simulink model "Quad_Tilt_Rotor_IdealModel"  (R2021b)
settings: Solver=FixedStepAuto  StartTime=0.0  StopTime=6  FixedStep=0.0001  RelTol=1e-3
values from neighbouring files (symbols this model uses):
  desired_initial_orientation = initial_orientation    [parameters_setting_Ideal.m]
  g = 9.8    [parameters_setting_Ideal.m]
  IB = [ 2.237568e-3  0               0 ... (first row only)    [parameters_setting_Ideal.m]
  initial_omega1 = initial_angular_vel1 * abs(initial_angular_vel1)    [parameters_setting_Ideal.m]
  initial_omega2 = initial_angular_vel2 * abs(initial_angular_vel2)    [parameters_setting_Ideal.m]
  initial_omega3 = initial_angular_vel3 * abs(initial_angular_vel3)    [parameters_setting_Ideal.m]
  initial_omega4 = initial_angular_vel4 * abs(initial_angular_vel4)    [parameters_setting_Ideal.m]
  initial_orientation = [ 1 0 0; 0 1 0; 0 0 1 ]    [parameters_setting_Ideal.m]
  Kf = 8.048e-6    (= 8.048e-06)    [parameters_setting_Ideal.m]
  Km = 2.423e-7    (= 2.423e-07)    [parameters_setting_Ideal.m]
  L = 0.1785    [parameters_setting_Ideal.m]
  lower_dalpha = -inf    [parameters_setting_Ideal.m]
  m = 0.429    [parameters_setting_Ideal.m]
  upper_dalpha = inf    [parameters_setting_Ideal.m]
libraries: vrlib x4, sharedutil x1, aerolibutil x1
settings Model: Creator=lucid  LastModifiedBy=lucid

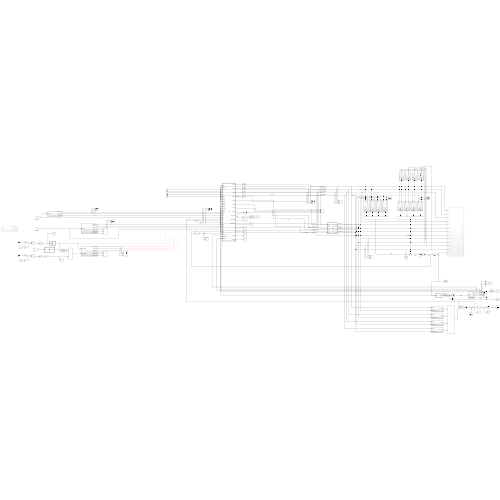
[thumbnail: Simulink's stored preview of the top-level diagram]
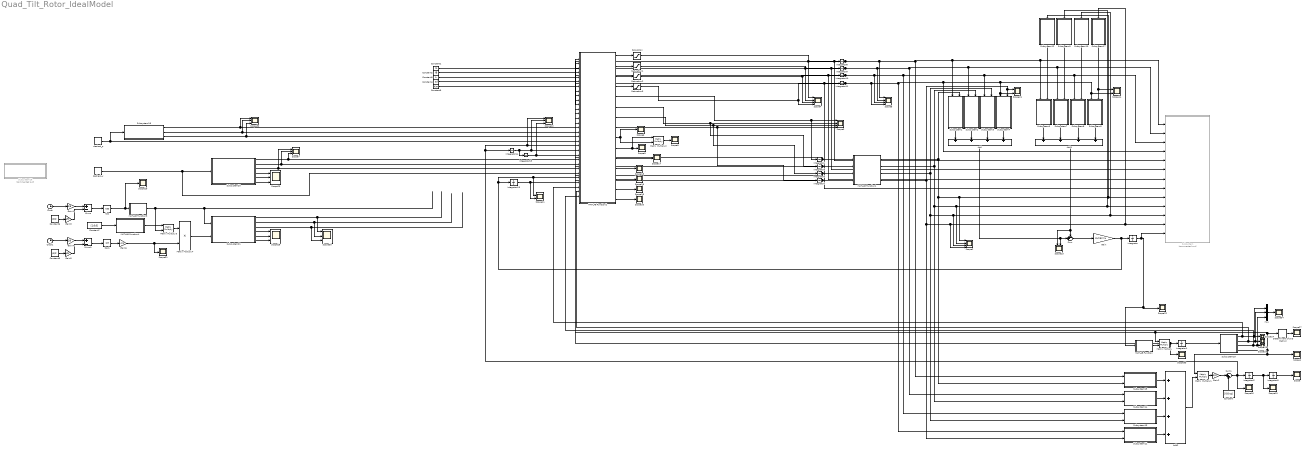
== system Quad_Tilt_Rotor_IdealModel ==
  Add : Sum  Inputs=++++
  Add1 : Sum  Inputs=++++
  Add2 : Sum  Inputs=++++
  Clock : Clock
  Clock1 : Clock
  Constant : Constant  Value=[0;0;-g]
  Constant1 : Constant  Value=m
  Constant2 : Constant  Value=IB
  Constant3 : Constant  Value=L
  Constant4 : Constant  Value=Kf
  Constant5 : Constant  Value=Km
  Constant6 : Constant  Value=pi/2
  Constant7 : Constant  Value=[1;0;0]
  Constant8 : Constant  Value=pi/2
  Cos : Trigonometry  Operator=cos
  Cos1 : Trigonometry
  Determinant of 3x3 Matrix2 : sharedutil/Determinant of 3x3 Matrix  aMode=aMode
      settings: SourceProductBaseCode=AE,PW,DR,MT,UV,VE
  Gain : Gain  Gain=inv(IB)  Multiplication=Matrix(K*u) (u vector)
  Gain{1,3..5} (4 alike) : Gain  Gain=1/6
  Gain2 : Gain  Gain=1/m
  Gain6 : Gain  Gain=-1/6
  Integrator{,2..3,8..11,13..15} (10 alike) : Integrator
  Integrator1 : Integrator  InitialCondition=initial_orientation
  Integrator4 : Integrator  InitialCondition=initial_omega1
  Integrator5 : Integrator  InitialCondition=initial_omega2
  Integrator6 : Integrator  InitialCondition=initial_omega3
  Integrator7 : Integrator  InitialCondition=initial_omega4
  MATLAB Function : MATLAB Function  TreatAsAtomicUnit=on
  MATLAB Function1 : MATLAB Function  TreatAsAtomicUnit=on
  MATLAB Function2 : MATLAB Function  TreatAsAtomicUnit=on
  MATLAB Function3 : MATLAB Function  TreatAsAtomicUnit=on
  MATLAB Function4 : MATLAB Function  TreatAsAtomicUnit=on
  Matrix Multiply{,1..3} (4 alike) : Product  Multiplication=Matrix(*)
  Matrix Multiply4 : Product
  Minus : Sum  Inputs=+-
  Minus1 : Sum  Inputs=+-
  Mux : Mux  Inputs=3
  Saturation{,1..3} (4 alike) : Saturate  UpperLimit=upper_dalpha  LowerLimit=lower_dalpha
  Scope{,1,6,8..10,15..20,22,24..27,29,31,33..34} (21 alike) : Scope
  Scope{11,13..14,21} (4 alike) : Scope  NumInputPorts=2
  Scope{7,12,23,28,30,32} (6 alike) : Scope  NumInputPorts=3
  Scope{2..5} (4 alike) : Scope  NumInputPorts=4
  Subsystem : Subsystem  Commented=on
  Subsystem1 : Subsystem
  Subsystem10 : Subsystem
  Subsystem11 : Subsystem
  Subsystem12 : Subsystem
  Subsystem13 : Subsystem
  Subsystem14 : Subsystem
  Subsystem15 : Subsystem
  Subsystem16 : Subsystem  Commented=on
  Subsystem17 : Subsystem
  Subsystem18 : Subsystem
  Subsystem19 : Subsystem
  Subsystem2 : Subsystem
  Subsystem20 : Subsystem
  Subsystem21 : Subsystem
  Subsystem3 : Subsystem
  Subsystem4 : Subsystem
  Subsystem5 : Subsystem
  Subsystem6 : Subsystem
  Subsystem7 : Subsystem
  Subsystem8 : Subsystem
  Subsystem9 : Subsystem
  Sum : Sum  Inputs=-+|
  Sum1 : Sum  Inputs=|++
  desired_p : Constant  Value=[0;0;0]
  desired_w : Constant  Value=[0;0;0]
  wires:
  Gain/1 -> Integrator13/1, Scope11/1, MATLAB Function2/27(dwB), Integrator/1  "dwB"
  Sum/1 -> Gain/1  "IB*dwB"
  Add/1 -> Scope13/2, Sum/2  "tauB"
  Add1/1 -> Sum/1, Scope13/1  "sumBtauP"
  Integrator/1 -> Subsystem/13(wB), MATLAB Function/1(w), Scope22/1  "wB"
  Subsystem1/1(tauB1) -> Add/1
  Subsystem2/1(tauB2) -> Add/2
  Subsystem3/1(tauB3) -> Add/3
  Subsystem4/1(tauB4) -> Add/4
  Subsystem5/1(BtauP4) -> Add1/4
  Subsystem6/1(BtauP1) -> Add1/1
  Subsystem7/1(BtauP2) -> Add1/2
  Subsystem8/1(BtauP3) -> Add1/3
  Subsystem17/1(tauP4) -> Subsystem5/2(tauP4), Scope14/1
  Subsystem12/1(tauP1) -> Subsystem6/2(tauP1)
  Subsystem9/1(tauP2) -> Subsystem7/2(tauP2)
  Subsystem10/1(tauP3) -> Subsystem8/2(tauP3)
  Integrator8/1 -> Scope5/1, Subsystem6/1(alpha1), Subsystem/1(alpha1), Subsystem1/1(alpha1), Subsystem15/1(alpha1), MATLAB Function2/8(alpha1)  "alpha1"
  Integrator9/1 -> Scope5/2, Subsystem7/1(alpha2), Subsystem/2(alpha2), Subsystem2/1(alpha2), Subsystem14/1(alpha2), MATLAB Function2/9(alpha2)  "alpha2"
  Integrator10/1 -> Scope5/3, Subsystem13/1(alpha3), Subsystem8/1(alpha3), Subsystem/3(alpha3), Subsystem3/1(alpha3), MATLAB Function2/10(alpha3)  "alpha3"
  Integrator11/1 -> Scope5/4, Scope14/2, Subsystem5/1(alpha4), Scope21/2, Subsystem4/1(alpha4), Subsystem/4(alpha4), Subsystem11/1(alpha4), MATLAB Function2/11(alpha4)  "alpha4"
  MATLAB Function1/1(angular_vel1) -> Subsystem15/2(angular_vel1), Scope2/1, Subsystem/9(angular_vel1), Subsystem12/1(Angular_vel1), Subsystem1/2(angular_vel1)  "angular_vel1"
  MATLAB Function1/2(angular_vel2) -> Subsystem14/2(angular_vel2), Scope2/2, Subsystem/10(angular_vel2), Subsystem9/1(Angular_vel2), Subsystem2/2(angular_vel2)  "angular_vel2"
  MATLAB Function1/3(angular_vel3) -> Subsystem13/2(angular_vel3), Scope2/3, Subsystem10/1(Angular_vel3), Subsystem/11(angular_vel3), Subsystem3/2(angular_vel3)  "angular_vel3"
  MATLAB Function1/4(angular_vel4) -> Subsystem11/2(angular_vel4), Scope2/4, Subsystem17/1(Angular_vel4), Subsystem/12(angular_vel4), Scope21/1, Subsystem4/2(angular_vel4)  "angular_vel4"
  Constant/1 -> Sum1/2
  Gain2/1 -> Sum1/1
  Integrator1/1 -> Subsystem19/1(WRB)  "WRB"
  Matrix Multiply/1 -> Scope33/1, Integrator1/1, MATLAB Function2/2(dWRB)  "dWRB"
  MATLAB Function/1(hat) -> Matrix Multiply/2
  Matrix Multiply1/1 -> Gain2/1
  Sum1/1 -> Scope16/1, Integrator14/1, Scope12/1, MATLAB Function2/20(ddp), Integrator2/1  "ddp"
  Add2/1 -> Matrix Multiply1/2
  Subsystem15/1(BTP1) -> Add2/1
  Subsystem14/1(BTP2) -> Add2/2
  Subsystem13/1(BTP3) -> Add2/3
  Subsystem11/1(BTP4) -> Add2/4
  Integrator2/1 -> Scope10/1, Integrator3/1  "dp"
  Integrator3/1 -> Scope/1  "p"
  Integrator4/1 -> MATLAB Function1/1(omega1), MATLAB Function2/12(omega1)
  Integrator5/1 -> MATLAB Function1/2(omega2), MATLAB Function2/13(omega2)
  Integrator6/1 -> MATLAB Function1/3(omega3), MATLAB Function2/14(omega3)
  Integrator7/1 -> MATLAB Function1/4(omega4), MATLAB Function2/15(omega4)
  MATLAB Function2/5(domega1) -> Integrator4/1, Scope3/1  "domega1"
  MATLAB Function2/6(domega2) -> Integrator5/1, Scope3/2  "domega2"
  MATLAB Function2/7(domega3) -> Integrator6/1, Scope3/3  "domega3"
  MATLAB Function2/8(domega4) -> Integrator7/1, Scope3/4  "domega4"
  MATLAB Function2/1(walpha1) -> Saturation/1  "walpha1"
  MATLAB Function2/2(walpha2) -> Saturation1/1  "walpha2"
  MATLAB Function2/3(walpha3) -> Saturation2/1  "walpha3"
  MATLAB Function2/4(walpha4) -> Saturation3/1  "walpha4"
  Constant1/1 -> MATLAB Function2/3(m)
  Constant2/1 -> MATLAB Function2/4(IB)
  Constant3/1 -> MATLAB Function2/5(L)
  Constant4/1 -> MATLAB Function2/6(Kf)
  Constant5/1 -> MATLAB Function2/7(Km)
  Integrator13/1 -> Scope11/2, MATLAB Function2/28(wB)  "wB"
  Integrator14/1 -> Integrator15/1, Scope12/2, MATLAB Function2/21(dp)
  Integrator15/1 -> Scope12/3, MATLAB Function2/22(p)
  desired_p/1 -> Subsystem18/1(desired_p), MATLAB Function2/19(pd)  "desired_p"
  desired_w/1 -> MATLAB Function2/26(wd), Subsystem20/1(desired_w)  "desired_w"
  Subsystem20/1(desired_WRB) -> MATLAB Function2/23(Rd), Scope7/3
  Subsystem20/2(desired_ddw) -> MATLAB Function2/24(ddwd), Scope7/2
  Subsystem20/3(desired_dw) -> MATLAB Function2/25(dwd), Scope7/1
  Subsystem18/1(desired_dddp) -> Scope32/1, MATLAB Function2/16(dddpd)
  Subsystem18/2(desired_ddp) -> Scope32/2, MATLAB Function2/17(ddpd)
  Subsystem18/3(desired_dp) -> Scope32/3, MATLAB Function2/18(dpd)
  MATLAB Function2/9(inverse_result) -> Scope6/1, Matrix Multiply2/2
  MATLAB Function2/10(ToBeInversed) -> Matrix Multiply2/1, Scope9/1
  Matrix Multiply2/1 -> Scope8/1
  MATLAB Function2/11(RankBeforeInv) -> Scope17/1
  MATLAB Function2/12(eR) -> Scope18/1
  MATLAB Function2/13(eP) -> Scope19/1
  MATLAB Function2/14(RankJR) -> Scope15/1
  MATLAB Function2/15(RankRight) -> Scope20/1
  Determinant of 3x3 Matrix2/1 -> Scope27/1
  Subsystem19/4(WRB_matrix) -> Scope1/1, Matrix Multiply1/1, MATLAB Function2/1(WRB), Matrix Multiply/1, Determinant of 3x3 Matrix2/1  "WRBm"
  Subsystem19/1(roll) -> MATLAB Function2/29(attitude_phi), Mux/1, Scope24/1
  Subsystem19/2(pitch) -> MATLAB Function2/30(attitude_theta), Mux/2, Scope25/1
  Saturation/1 -> Scope4/1, Subsystem/5(dalpha1), Integrator8/1
  Saturation1/1 -> Scope4/2, Subsystem/6(dalpha2), Integrator9/1
  Saturation2/1 -> Scope4/3, Integrator10/1, Subsystem/7(dalpha3)
  Saturation3/1 -> Scope4/4, Integrator11/1, Subsystem/8(dalpha4)
  Subsystem19/3(yaw) -> MATLAB Function2/31(attitude_psi), Mux/3, Scope26/1
  Subsystem20/4(desired_roll) -> Scope23/1
  Subsystem20/5(desired_pitch) -> Scope23/2
  Subsystem20/6(desired_yaw) -> Scope23/3
  Subsystem21/4(desired_roll) -> Scope28/1
  Subsystem21/5(desired_pitch) -> Scope28/2
  Subsystem21/6(desired_yaw) -> Scope28/3
  MATLAB Function3/1(R) -> Matrix Multiply3/2, Subsystem21/1(desired_wRb)
  Subsystem21/3(desired_w) -> Scope30/3
  Subsystem21/2(desired_dw) -> Scope30/2
  Subsystem21/1(desired_ddw) -> Scope30/1
  Cos/1 -> Scope29/1, MATLAB Function3/1(theta)
  Minus/1 -> Cos/1
  Constant6/1 -> Gain3/1
  Gain1/1 -> Minus/1
  Clock/1 -> Gain1/1
  Gain3/1 -> Minus/2
  Constant7/1 -> MATLAB Function4/1(vector)
  MATLAB Function4/1(skewed) -> Matrix Multiply3/1
  Matrix Multiply3/1 -> Matrix Multiply4/1
  Matrix Multiply4/1 -> Subsystem21/2(desired_dwRb)
  Gain6/1 -> Scope31/1, Matrix Multiply4/2
  Gain5/1 -> Minus1/2
  Clock1/1 -> Gain4/1
  Gain4/1 -> Minus1/1
  Constant8/1 -> Gain5/1
  Minus1/1 -> Cos1/1
  Cos1/1 -> Gain6/1
  Mux/1 -> Scope34/1

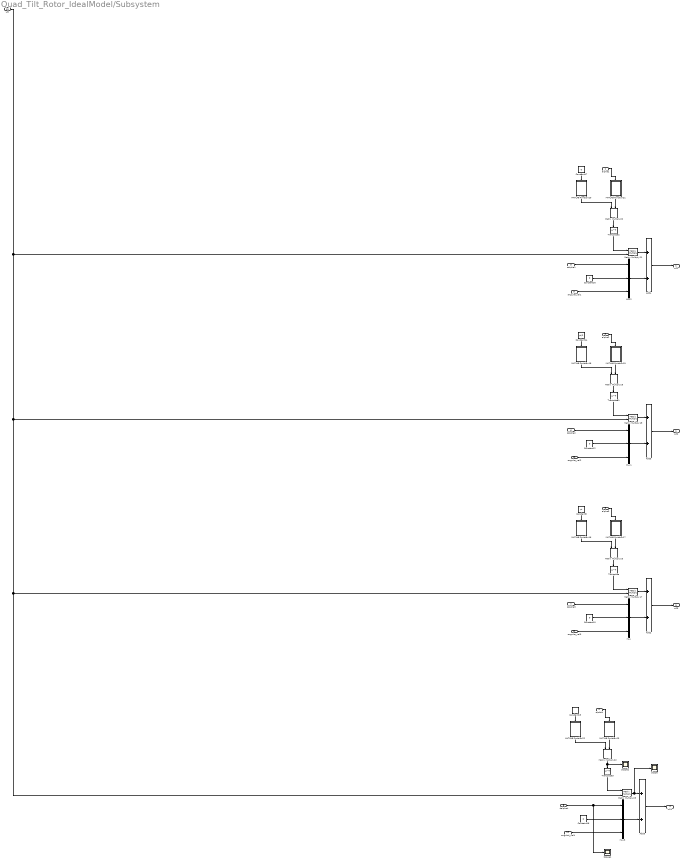
== system Quad_Tilt_Rotor_IdealModel/Subsystem ==
  alpha1 : Inport
  alpha2 : Inport  Port=2
  alpha3 : Inport  Port=3
  alpha4 : Inport  Port=4
  dalpha1 : Inport  Port=5
  dalpha2 : Inport  Port=6
  dalpha3 : Inport  Port=7
  dalpha4 : Inport  Port=8
  angular_vel1 : Inport  Port=9
  angular_vel2 : Inport  Port=10
  angular_vel3 : Inport  Port=11
  angular_vel4 : Inport  Port=12
  wB : Inport  Port=13
  Add{2..5} (4 alike) : Sum
  Constant{10,12,16..18} (5 alike) : Constant  Value=0
  Constant14 : Constant  Value=pi/2
  Constant19 : Constant  Value=3*pi/2
  Constant8 : Constant  Value=pi
  MATLAB Function16 : MATLAB Function  TreatAsAtomicUnit=on
  MATLAB Function17 : MATLAB Function  TreatAsAtomicUnit=on
  MATLAB Function18 : MATLAB Function  TreatAsAtomicUnit=on
  MATLAB Function19 : MATLAB Function  TreatAsAtomicUnit=on
  MATLAB Function20 : MATLAB Function  TreatAsAtomicUnit=on
  MATLAB Function21 : MATLAB Function  TreatAsAtomicUnit=on
  MATLAB Function22 : MATLAB Function  TreatAsAtomicUnit=on
  MATLAB Function23 : MATLAB Function  TreatAsAtomicUnit=on
  Matrix Multiply{16..23} (8 alike) : Product  Multiplication=Matrix(*)
  Mux{,1..3} (4 alike) : Mux  Inputs=3
  Scope : Scope
  Scope1 : Scope
  Scope2 : Scope
  Transpose{,1..3} (4 alike) : Math  Operator=transpose  SaturateOnIntegerOverflow=on
  wP1 : Outport
  wP2 : Outport  Port=2
  wP3 : Outport  Port=3
  wP4 : Outport  Port=4
  wires:
  Matrix Multiply19/1 -> Add3/1
  Constant10/1 -> Mux/2
  Transpose3/1 -> Matrix Multiply23/1
  alpha3/1 -> MATLAB Function17/1(theta)
  wB/1 -> Matrix Multiply19/2, Matrix Multiply23/2, Matrix Multiply17/2, Matrix Multiply21/2
  alpha2/1 -> MATLAB Function19/1(theta)
  Mux/1 -> Add2/2
  Constant19/1 -> MATLAB Function22/1(theta)
  Constant18/1 -> Mux3/2
  dalpha3/1 -> Mux/1  "dalpha3"
  Matrix Multiply23/1 -> Scope/1, Add5/1
  Matrix Multiply16/1 -> Transpose/1
  MATLAB Function20/1(R) -> Matrix Multiply20/1
  angular_vel2/1 -> Mux1/3
  Mux3/1 -> Add5/2
  alpha1/1 -> MATLAB Function21/1(theta)
  MATLAB Function21/1(R) -> Matrix Multiply20/2
  Constant17/1 -> MATLAB Function20/1(theta)
  Add5/1 -> wP4/1  "wP4"
  Matrix Multiply20/1 -> Transpose2/1
  dalpha4/1 -> Scope1/1, Mux3/1  "dalpha4"
  Matrix Multiply21/1 -> Add4/1
  MATLAB Function19/1(R) -> Matrix Multiply18/2
  dalpha1/1 -> Mux2/1  "dalpha1"
  Transpose1/1 -> Matrix Multiply19/1
  Add4/1 -> wP1/1  "wP1"
  Mux2/1 -> Add4/2
  Transpose2/1 -> Matrix Multiply21/1
  MATLAB Function16/1(R) -> Matrix Multiply16/1
  Constant16/1 -> Mux2/2
  angular_vel1/1 -> Mux2/3
  Matrix Multiply18/1 -> Transpose1/1
  Constant14/1 -> MATLAB Function18/1(theta)
  angular_vel4/1 -> Mux3/3
  Constant12/1 -> Mux1/2
  MATLAB Function23/1(R) -> Matrix Multiply22/2
  alpha4/1 -> MATLAB Function23/1(theta)
  Mux1/1 -> Add3/2
  MATLAB Function22/1(R) -> Matrix Multiply22/1
  Add2/1 -> wP3/1  "wP3"
  MATLAB Function18/1(R) -> Matrix Multiply18/1
  dalpha2/1 -> Mux1/1  "dalpha2"
  Transpose/1 -> Matrix Multiply17/1
  Matrix Multiply22/1 -> Scope2/1, Transpose3/1
  Constant8/1 -> MATLAB Function16/1(theta)
  Matrix Multiply17/1 -> Add2/1
  MATLAB Function17/1(R) -> Matrix Multiply16/2
  angular_vel3/1 -> Mux/3
  Add3/1 -> wP2/1  "wP2"

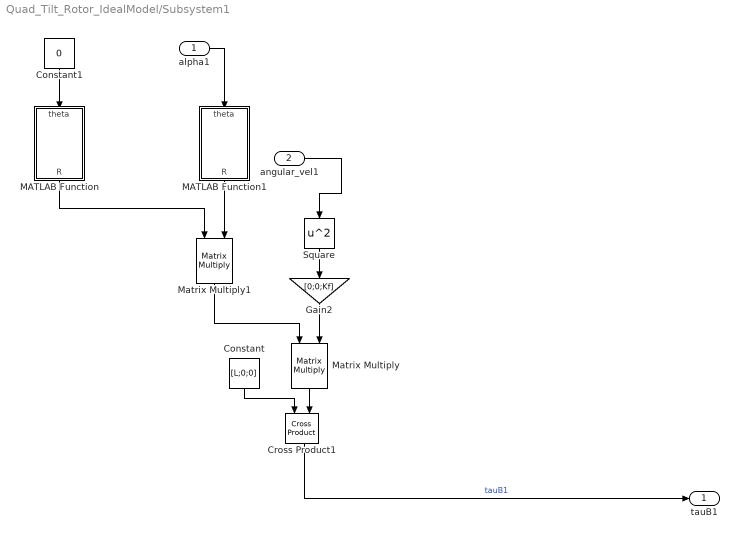
== system Quad_Tilt_Rotor_IdealModel/Subsystem1 ==
  alpha1 : Inport
  angular_vel1 : Inport  Port=2
  Constant : Constant  Value=[L;0;0]
  Constant1 : Constant  Value=0
  Cross Product1 : vrlib/Utilities/Cross Product
  Gain2 : Gain  Gain=[0;0;Kf]
  MATLAB Function : MATLAB Function  TreatAsAtomicUnit=on
  MATLAB Function1 : MATLAB Function  TreatAsAtomicUnit=on
  Matrix Multiply : Product  Multiplication=Matrix(*)
  Matrix Multiply1 : Product  Multiplication=Matrix(*)
  Square : Math  Operator=square  SaturateOnIntegerOverflow=on
  tauB1 : Outport
  wires:
  Constant1/1 -> MATLAB Function/1(theta)
  Matrix Multiply/1 -> Cross Product1/2
  MATLAB Function1/1(R) -> Matrix Multiply1/2
  Constant/1 -> Cross Product1/1
  MATLAB Function/1(R) -> Matrix Multiply1/1
  Square/1 -> Gain2/1
  Gain2/1 -> Matrix Multiply/2
  Matrix Multiply1/1 -> Matrix Multiply/1
  angular_vel1/1 -> Square/1
  Cross Product1/1 -> tauB1/1  "tauB1"
  alpha1/1 -> MATLAB Function1/1(theta)

== system Quad_Tilt_Rotor_IdealModel/Subsystem10 ==
  Angular_vel3 : Inport
  Gain : Gain  Gain=-1
  Subsystem15 : Subsystem
  tauP3 : Outport
  wires:
  Angular_vel3/1 -> Subsystem15/1(Angular_vel3)
  Gain/1 -> tauP3/1  "tauP3"
  Subsystem15/1(tauext3) -> Gain/1

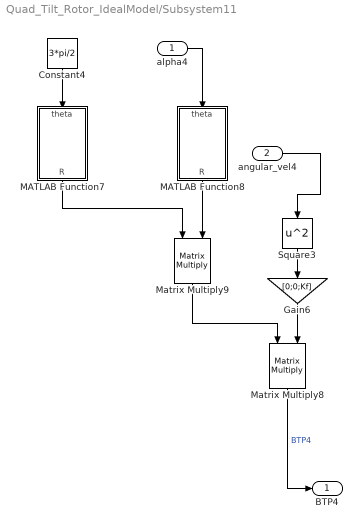
== system Quad_Tilt_Rotor_IdealModel/Subsystem11 ==
  alpha4 : Inport
  angular_vel4 : Inport  Port=2
  Constant4 : Constant  Value=3*pi/2
  Gain6 : Gain  Gain=[0;0;Kf]
  MATLAB Function7 : MATLAB Function  TreatAsAtomicUnit=on
  MATLAB Function8 : MATLAB Function  TreatAsAtomicUnit=on
  Matrix Multiply8 : Product  Multiplication=Matrix(*)
  Matrix Multiply9 : Product  Multiplication=Matrix(*)
  Square3 : Math  Operator=square  SaturateOnIntegerOverflow=on
  BTP4 : Outport
  wires:
  Square3/1 -> Gain6/1
  angular_vel4/1 -> Square3/1
  MATLAB Function8/1(R) -> Matrix Multiply9/2
  MATLAB Function7/1(R) -> Matrix Multiply9/1
  Constant4/1 -> MATLAB Function7/1(theta)
  Matrix Multiply8/1 -> BTP4/1  "BTP4"
  Gain6/1 -> Matrix Multiply8/2
  Matrix Multiply9/1 -> Matrix Multiply8/1
  alpha4/1 -> MATLAB Function8/1(theta)

== system Quad_Tilt_Rotor_IdealModel/Subsystem12 ==
  Angular_vel1 : Inport
  Gain : Gain  Gain=-1
  Subsystem13 : Subsystem
  tauP1 : Outport
  wires:
  Angular_vel1/1 -> Subsystem13/1(Angular_vel1)
  Subsystem13/1(tauext1) -> Gain/1
  Gain/1 -> tauP1/1  "tauP1"

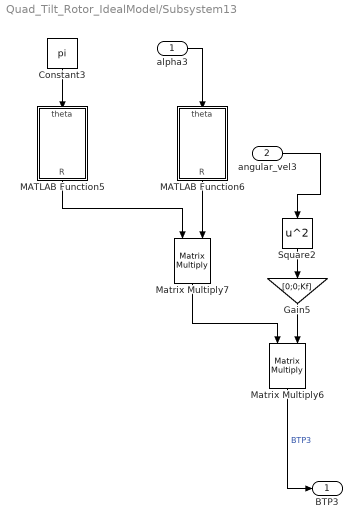
== system Quad_Tilt_Rotor_IdealModel/Subsystem13 ==
  alpha3 : Inport
  angular_vel3 : Inport  Port=2
  Constant3 : Constant  Value=pi
  Gain5 : Gain  Gain=[0;0;Kf]
  MATLAB Function5 : MATLAB Function  TreatAsAtomicUnit=on
  MATLAB Function6 : MATLAB Function  TreatAsAtomicUnit=on
  Matrix Multiply6 : Product  Multiplication=Matrix(*)
  Matrix Multiply7 : Product  Multiplication=Matrix(*)
  Square2 : Math  Operator=square  SaturateOnIntegerOverflow=on
  BTP3 : Outport
  wires:
  Gain5/1 -> Matrix Multiply6/2
  alpha3/1 -> MATLAB Function6/1(theta)
  Constant3/1 -> MATLAB Function5/1(theta)
  Matrix Multiply7/1 -> Matrix Multiply6/1
  Square2/1 -> Gain5/1
  Matrix Multiply6/1 -> BTP3/1  "BTP3"
  MATLAB Function5/1(R) -> Matrix Multiply7/1
  MATLAB Function6/1(R) -> Matrix Multiply7/2
  angular_vel3/1 -> Square2/1

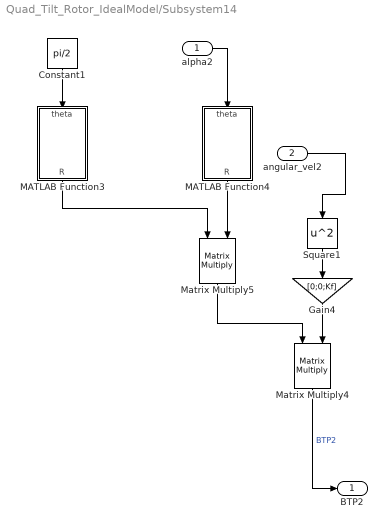
== system Quad_Tilt_Rotor_IdealModel/Subsystem14 ==
  alpha2 : Inport
  angular_vel2 : Inport  Port=2
  Constant1 : Constant  Value=pi/2
  Gain4 : Gain  Gain=[0;0;Kf]
  MATLAB Function3 : MATLAB Function  TreatAsAtomicUnit=on
  MATLAB Function4 : MATLAB Function  TreatAsAtomicUnit=on
  Matrix Multiply4 : Product  Multiplication=Matrix(*)
  Matrix Multiply5 : Product  Multiplication=Matrix(*)
  Square1 : Math  Operator=square  SaturateOnIntegerOverflow=on
  BTP2 : Outport
  wires:
  Matrix Multiply5/1 -> Matrix Multiply4/1
  MATLAB Function3/1(R) -> Matrix Multiply5/1
  Matrix Multiply4/1 -> BTP2/1  "BTP2"
  MATLAB Function4/1(R) -> Matrix Multiply5/2
  Square1/1 -> Gain4/1
  angular_vel2/1 -> Square1/1
  Constant1/1 -> MATLAB Function3/1(theta)
  Gain4/1 -> Matrix Multiply4/2
  alpha2/1 -> MATLAB Function4/1(theta)

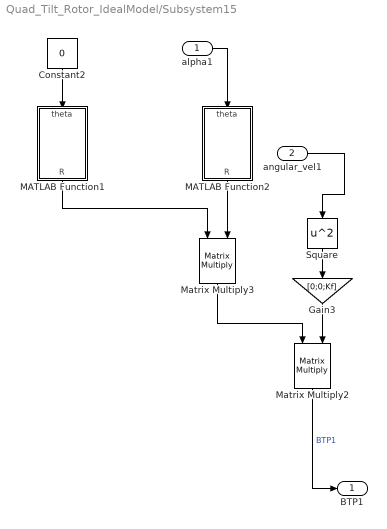
== system Quad_Tilt_Rotor_IdealModel/Subsystem15 ==
  alpha1 : Inport
  angular_vel1 : Inport  Port=2
  Constant2 : Constant  Value=0
  Gain3 : Gain  Gain=[0;0;Kf]
  MATLAB Function1 : MATLAB Function  TreatAsAtomicUnit=on
  MATLAB Function2 : MATLAB Function  TreatAsAtomicUnit=on
  Matrix Multiply2 : Product  Multiplication=Matrix(*)
  Matrix Multiply3 : Product  Multiplication=Matrix(*)
  Square : Math  Operator=square  SaturateOnIntegerOverflow=on
  BTP1 : Outport
  wires:
  Gain3/1 -> Matrix Multiply2/2
  MATLAB Function2/1(R) -> Matrix Multiply3/2
  angular_vel1/1 -> Square/1
  Square/1 -> Gain3/1
  Constant2/1 -> MATLAB Function1/1(theta)
  MATLAB Function1/1(R) -> Matrix Multiply3/1
  Matrix Multiply3/1 -> Matrix Multiply2/1
  alpha1/1 -> MATLAB Function2/1(theta)
  Matrix Multiply2/1 -> BTP1/1  "BTP1"

== system Quad_Tilt_Rotor_IdealModel/Subsystem16 ==
  desired_w : Inport
  Derivative3 : Derivative
  Derivative4 : Derivative
  Integrator16 : Integrator  InitialCondition=desired_initial_orientation
  MATLAB Function3 : MATLAB Function  TreatAsAtomicUnit=on
  Matrix Multiply2 : Product  Multiplication=Matrix(*)
  Scope : Scope
  desired_WRB : Outport
  desired_ddw : Outport  Port=2
  desired_dw : Outport  Port=3
  wires:
  Derivative3/1 -> desired_dw/1, Derivative4/1  "desired_dw"
  Derivative4/1 -> desired_ddw/1  "desired_ddw"
  Matrix Multiply2/1 -> Integrator16/1  "desired_dWRB"
  Integrator16/1 -> Scope/1, desired_WRB/1, Matrix Multiply2/1  "desired_WRB"
  MATLAB Function3/1(hat) -> Matrix Multiply2/2
  desired_w/1 -> Derivative3/1, MATLAB Function3/1(w)

== system Quad_Tilt_Rotor_IdealModel/Subsystem17 ==
  Angular_vel4 : Inport
  Gain : Gain  Gain=-1
  Subsystem16 : Subsystem
  tauP4 : Outport
  wires:
  Angular_vel4/1 -> Subsystem16/1(Angular_vel4)
  Gain/1 -> tauP4/1  "tauP4"
  Subsystem16/1(tauext4) -> Gain/1

== system Quad_Tilt_Rotor_IdealModel/Subsystem18 ==
  desired_p : Inport
  Derivative : Derivative
  Derivative1 : Derivative
  Derivative2 : Derivative
  desired_dddp : Outport
  desired_ddp : Outport  Port=2
  desired_dp : Outport  Port=3
  wires:
  Derivative/1 -> desired_dp/1, Derivative1/1  "desired_dp"
  desired_p/1 -> Derivative/1
  Derivative1/1 -> desired_ddp/1, Derivative2/1  "desired_ddp"
  Derivative2/1 -> desired_dddp/1  "desired_dddp"

== system Quad_Tilt_Rotor_IdealModel/Subsystem19 ==
  WRB : Inport
  to rotm : MATLAB Function  TreatAsAtomicUnit=on
  to rpy : MATLAB Function  TreatAsAtomicUnit=on
  roll : Outport
  pitch : Outport  Port=2
  yaw : Outport  Port=3
  WRB_matrix : Outport  Port=4
  wires:
  to rpy/3(roll) -> roll/1, to rotm/3(phi)
  to rpy/2(pitch) -> pitch/1, to rotm/2(theta)
  WRB/1 -> to rpy/1(rotation_matrix)
  to rpy/1(yaw) -> to rotm/1(psi), yaw/1
  to rotm/1(rotm) -> WRB_matrix/1  "WRB"

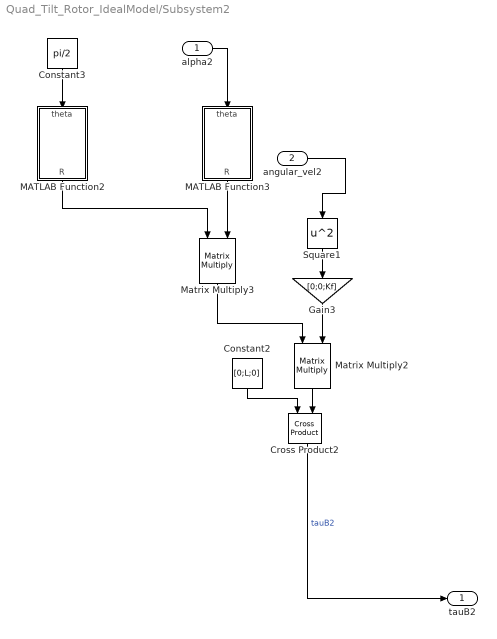
== system Quad_Tilt_Rotor_IdealModel/Subsystem2 ==
  alpha2 : Inport
  angular_vel2 : Inport  Port=2
  Constant2 : Constant  Value=[0;L;0]
  Constant3 : Constant  Value=pi/2
  Cross Product2 : vrlib/Utilities/Cross Product
  Gain3 : Gain  Gain=[0;0;Kf]
  MATLAB Function2 : MATLAB Function  TreatAsAtomicUnit=on
  MATLAB Function3 : MATLAB Function  TreatAsAtomicUnit=on
  Matrix Multiply2 : Product  Multiplication=Matrix(*)
  Matrix Multiply3 : Product  Multiplication=Matrix(*)
  Square1 : Math  Operator=square  SaturateOnIntegerOverflow=on
  tauB2 : Outport
  wires:
  angular_vel2/1 -> Square1/1
  Constant2/1 -> Cross Product2/1
  MATLAB Function3/1(R) -> Matrix Multiply3/2
  MATLAB Function2/1(R) -> Matrix Multiply3/1
  Gain3/1 -> Matrix Multiply2/2
  Square1/1 -> Gain3/1
  Matrix Multiply3/1 -> Matrix Multiply2/1
  Constant3/1 -> MATLAB Function2/1(theta)
  Matrix Multiply2/1 -> Cross Product2/2
  alpha2/1 -> MATLAB Function3/1(theta)
  Cross Product2/1 -> tauB2/1  "tauB2"

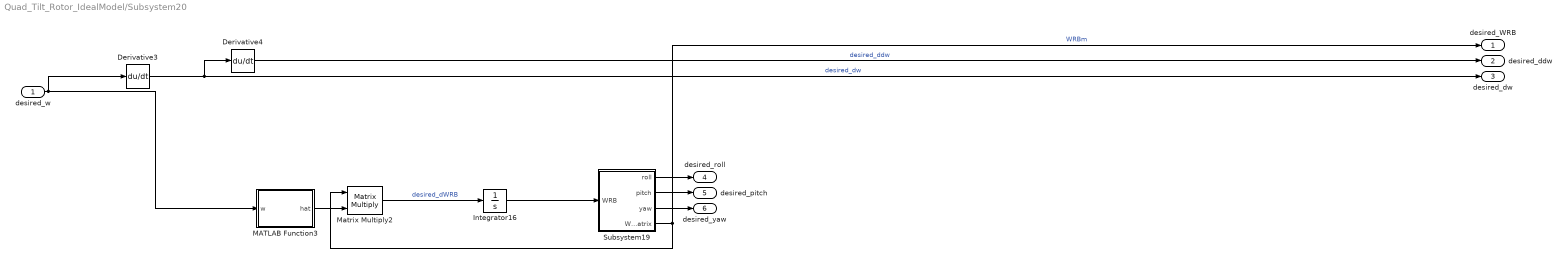
== system Quad_Tilt_Rotor_IdealModel/Subsystem20 ==
  desired_w : Inport
  Derivative3 : Derivative
  Derivative4 : Derivative
  Integrator16 : Integrator  InitialCondition=desired_initial_orientation
  MATLAB Function3 : MATLAB Function  TreatAsAtomicUnit=on
  Matrix Multiply2 : Product  Multiplication=Matrix(*)
  Subsystem19 : Subsystem
  desired_WRB : Outport
  desired_ddw : Outport  Port=2
  desired_dw : Outport  Port=3
  desired_roll : Outport  Port=4
  desired_pitch : Outport  Port=5
  desired_yaw : Outport  Port=6
  wires:
  Derivative3/1 -> desired_dw/1, Derivative4/1  "desired_dw"
  Derivative4/1 -> desired_ddw/1  "desired_ddw"
  Matrix Multiply2/1 -> Integrator16/1  "desired_dWRB"
  Integrator16/1 -> Subsystem19/1(WRB)
  MATLAB Function3/1(hat) -> Matrix Multiply2/2
  desired_w/1 -> Derivative3/1, MATLAB Function3/1(w)
  Subsystem19/4(WRB_matrix) -> desired_WRB/1, Matrix Multiply2/1  "WRBm"
  Subsystem19/1(roll) -> desired_roll/1
  Subsystem19/2(pitch) -> desired_pitch/1
  Subsystem19/3(yaw) -> desired_yaw/1

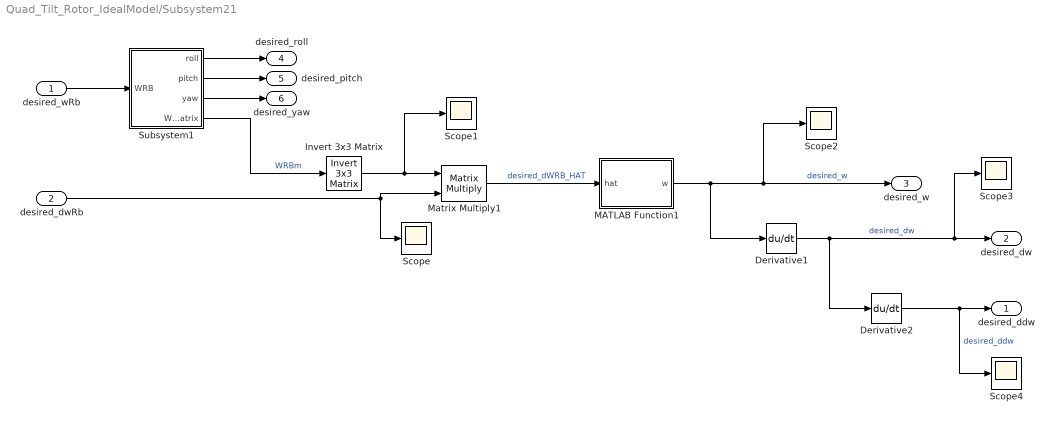
== system Quad_Tilt_Rotor_IdealModel/Subsystem21 ==
  desired_wRb : Inport
  desired_dwRb : Inport  Port=2
  Derivative1 : Derivative
  Derivative2 : Derivative
  Invert 3x3 Matrix : aerolibutil/Invert  3x3 Matrix
  MATLAB Function1 : MATLAB Function  TreatAsAtomicUnit=on
  Matrix Multiply1 : Product  Multiplication=Matrix(*)
  Scope{,1..4} (5 alike) : Scope
  Subsystem1 : Subsystem
  desired_ddw : Outport
  desired_dw : Outport  Port=2
  desired_w : Outport  Port=3
  desired_roll : Outport  Port=4
  desired_pitch : Outport  Port=5
  desired_yaw : Outport  Port=6
  wires:
  desired_wRb/1 -> Subsystem1/1(WRB)
  Matrix Multiply1/1 -> MATLAB Function1/1(hat)  "desired_dWRB_HAT"
  Subsystem1/4(WRB_matrix) -> Invert 3x3 Matrix/1  "WRBm"
  desired_dwRb/1 -> Scope/1, Matrix Multiply1/2
  Invert 3x3 Matrix/1 -> Scope1/1, Matrix Multiply1/1
  MATLAB Function1/1(w) -> Scope2/1, desired_w/1, Derivative1/1  "desired_w"
  Derivative1/1 -> Scope3/1, desired_dw/1, Derivative2/1  "desired_dw"
  Derivative2/1 -> Scope4/1, desired_ddw/1  "desired_ddw"
  Subsystem1/1(roll) -> desired_roll/1
  Subsystem1/2(pitch) -> desired_pitch/1
  Subsystem1/3(yaw) -> desired_yaw/1

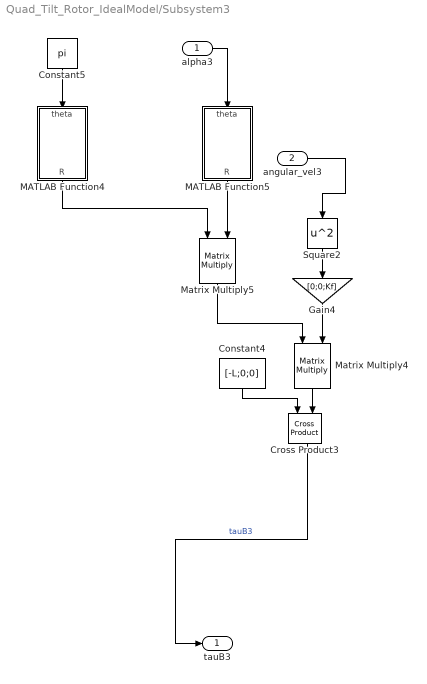
== system Quad_Tilt_Rotor_IdealModel/Subsystem3 ==
  alpha3 : Inport
  angular_vel3 : Inport  Port=2
  Constant4 : Constant  Value=[-L;0;0]
  Constant5 : Constant  Value=pi
  Cross Product3 : vrlib/Utilities/Cross Product
  Gain4 : Gain  Gain=[0;0;Kf]
  MATLAB Function4 : MATLAB Function  TreatAsAtomicUnit=on
  MATLAB Function5 : MATLAB Function  TreatAsAtomicUnit=on
  Matrix Multiply4 : Product  Multiplication=Matrix(*)
  Matrix Multiply5 : Product  Multiplication=Matrix(*)
  Square2 : Math  Operator=square  SaturateOnIntegerOverflow=on
  tauB3 : Outport
  wires:
  Matrix Multiply4/1 -> Cross Product3/2
  Square2/1 -> Gain4/1
  Matrix Multiply5/1 -> Matrix Multiply4/1
  Constant4/1 -> Cross Product3/1
  Gain4/1 -> Matrix Multiply4/2
  Constant5/1 -> MATLAB Function4/1(theta)
  MATLAB Function4/1(R) -> Matrix Multiply5/1
  MATLAB Function5/1(R) -> Matrix Multiply5/2
  alpha3/1 -> MATLAB Function5/1(theta)
  angular_vel3/1 -> Square2/1
  Cross Product3/1 -> tauB3/1  "tauB3"

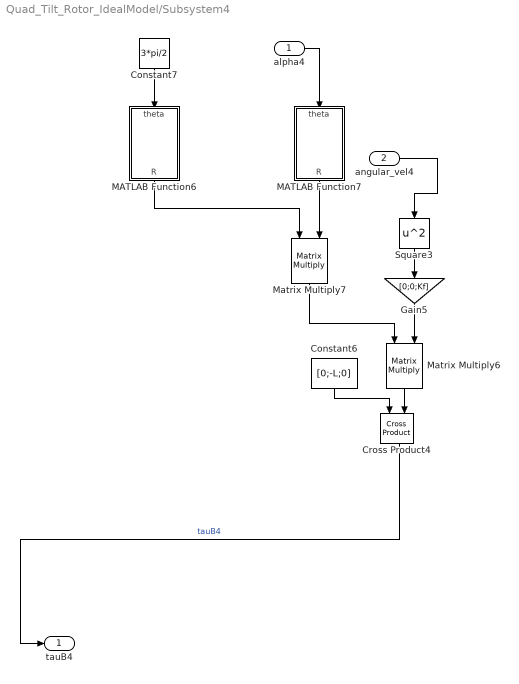
== system Quad_Tilt_Rotor_IdealModel/Subsystem4 ==
  alpha4 : Inport
  angular_vel4 : Inport  Port=2
  Constant6 : Constant  Value=[0;-L;0]
  Constant7 : Constant  Value=3*pi/2
  Cross Product4 : vrlib/Utilities/Cross Product
  Gain5 : Gain  Gain=[0;0;Kf]
  MATLAB Function6 : MATLAB Function  TreatAsAtomicUnit=on
  MATLAB Function7 : MATLAB Function  TreatAsAtomicUnit=on
  Matrix Multiply6 : Product  Multiplication=Matrix(*)
  Matrix Multiply7 : Product  Multiplication=Matrix(*)
  Square3 : Math  Operator=square  SaturateOnIntegerOverflow=on
  tauB4 : Outport
  wires:
  Gain5/1 -> Matrix Multiply6/2
  Constant7/1 -> MATLAB Function6/1(theta)
  Matrix Multiply6/1 -> Cross Product4/2
  alpha4/1 -> MATLAB Function7/1(theta)
  MATLAB Function6/1(R) -> Matrix Multiply7/1
  MATLAB Function7/1(R) -> Matrix Multiply7/2
  Constant6/1 -> Cross Product4/1
  Square3/1 -> Gain5/1
  Matrix Multiply7/1 -> Matrix Multiply6/1
  Cross Product4/1 -> tauB4/1  "tauB4"
  angular_vel4/1 -> Square3/1

== system Quad_Tilt_Rotor_IdealModel/Subsystem5 ==
  alpha4 : Inport
  tauP4 : Inport  Port=2
  Constant15 : Constant  Value=3*pi/2
  MATLAB Function14 : MATLAB Function  TreatAsAtomicUnit=on
  MATLAB Function15 : MATLAB Function  TreatAsAtomicUnit=on
  Matrix Multiply14 : Product  Multiplication=Matrix(*)
  Matrix Multiply15 : Product  Multiplication=Matrix(*)
  BtauP4 : Outport
  wires:
  Matrix Multiply15/1 -> Matrix Multiply14/1
  MATLAB Function15/1(R) -> Matrix Multiply15/2
  MATLAB Function14/1(R) -> Matrix Multiply15/1
  Matrix Multiply14/1 -> BtauP4/1  "BtauP4"
  Constant15/1 -> MATLAB Function14/1(theta)
  tauP4/1 -> Matrix Multiply14/2
  alpha4/1 -> MATLAB Function15/1(theta)

== system Quad_Tilt_Rotor_IdealModel/Subsystem6 ==
  alpha1 : Inport
  tauP1 : Inport  Port=2
  Constant9 : Constant  Value=0
  MATLAB Function8 : MATLAB Function  TreatAsAtomicUnit=on
  MATLAB Function9 : MATLAB Function  TreatAsAtomicUnit=on
  Matrix Multiply8 : Product  Multiplication=Matrix(*)
  Matrix Multiply9 : Product  Multiplication=Matrix(*)
  BtauP1 : Outport
  wires:
  tauP1/1 -> Matrix Multiply8/2
  Constant9/1 -> MATLAB Function8/1(theta)
  MATLAB Function8/1(R) -> Matrix Multiply9/1
  MATLAB Function9/1(R) -> Matrix Multiply9/2
  alpha1/1 -> MATLAB Function9/1(theta)
  Matrix Multiply9/1 -> Matrix Multiply8/1
  Matrix Multiply8/1 -> BtauP1/1  "BtauP1"

== system Quad_Tilt_Rotor_IdealModel/Subsystem7 ==
  alpha2 : Inport
  tauP2 : Inport  Port=2
  Constant11 : Constant  Value=pi/2
  MATLAB Function10 : MATLAB Function  TreatAsAtomicUnit=on
  MATLAB Function11 : MATLAB Function  TreatAsAtomicUnit=on
  Matrix Multiply10 : Product  Multiplication=Matrix(*)
  Matrix Multiply11 : Product  Multiplication=Matrix(*)
  BtauP2 : Outport
  wires:
  Constant11/1 -> MATLAB Function10/1(theta)
  Matrix Multiply11/1 -> Matrix Multiply10/1
  MATLAB Function10/1(R) -> Matrix Multiply11/1
  tauP2/1 -> Matrix Multiply10/2
  MATLAB Function11/1(R) -> Matrix Multiply11/2
  Matrix Multiply10/1 -> BtauP2/1  "BtauP2"
  alpha2/1 -> MATLAB Function11/1(theta)

== system Quad_Tilt_Rotor_IdealModel/Subsystem8 ==
  alpha3 : Inport
  tauP3 : Inport  Port=2
  Constant13 : Constant  Value=pi
  MATLAB Function12 : MATLAB Function  TreatAsAtomicUnit=on
  MATLAB Function13 : MATLAB Function  TreatAsAtomicUnit=on
  Matrix Multiply12 : Product  Multiplication=Matrix(*)
  Matrix Multiply13 : Product  Multiplication=Matrix(*)
  BtauP3 : Outport
  wires:
  Constant13/1 -> MATLAB Function12/1(theta)
  Matrix Multiply13/1 -> Matrix Multiply12/1
  alpha3/1 -> MATLAB Function13/1(theta)
  MATLAB Function12/1(R) -> Matrix Multiply13/1
  MATLAB Function13/1(R) -> Matrix Multiply13/2
  tauP3/1 -> Matrix Multiply12/2
  Matrix Multiply12/1 -> BtauP3/1  "BtauP3"

== system Quad_Tilt_Rotor_IdealModel/Subsystem9 ==
  Angular_vel2 : Inport
  Gain : Gain  Gain=-1
  Subsystem14 : Subsystem
  tauP2 : Outport
  wires:
  Angular_vel2/1 -> Subsystem14/1(Angular_vel2)
  Gain/1 -> tauP2/1  "tauP2"
  Subsystem14/1(tauext2) -> Gain/1

== system Quad_Tilt_Rotor_IdealModel/Subsystem10/Subsystem15 ==
  Angular_vel3 : Inport
  Abs : Abs
  Gain2 : Gain  Gain=[0;0;-Km]  Multiplication=Matrix(K*u) (u vector)
  Matrix Multiply : Product  Multiplication=Matrix(*)
  tauext3 : Outport
  wires:
  Matrix Multiply/1 -> Gain2/1
  Gain2/1 -> tauext3/1
  Abs/1 -> Matrix Multiply/2  "abs(Angular_vel3)"
  Angular_vel3/1 -> Matrix Multiply/1, Abs/1  "Angular_vel3"

== system Quad_Tilt_Rotor_IdealModel/Subsystem12/Subsystem13 ==
  Angular_vel1 : Inport
  Abs : Abs
  Gain2 : Gain  Gain=[0;0;-Km]  Multiplication=Matrix(K*u) (u vector)
  Matrix Multiply : Product  Multiplication=Matrix(*)
  tauext1 : Outport
  wires:
  Matrix Multiply/1 -> Gain2/1
  Gain2/1 -> tauext1/1
  Abs/1 -> Matrix Multiply/2  "abs(Angular_vel1Z)"
  Angular_vel1/1 -> Matrix Multiply/1, Abs/1

== system Quad_Tilt_Rotor_IdealModel/Subsystem17/Subsystem16 ==
  Angular_vel4 : Inport
  Abs : Abs
  Gain2 : Gain  Gain=[0;0;-Km]  Multiplication=Matrix(K*u) (u vector)
  Matrix Multiply : Product  Multiplication=Matrix(*)
  tauext4 : Outport
  wires:
  Angular_vel4/1 -> Abs/1, Matrix Multiply/1  "Angular_vel4"
  Abs/1 -> Matrix Multiply/2  "abs(Angular_vel4)"
  Gain2/1 -> tauext4/1
  Matrix Multiply/1 -> Gain2/1

== system Quad_Tilt_Rotor_IdealModel/Subsystem20/Subsystem19 ==
  WRB : Inport
  to rotm : MATLAB Function  TreatAsAtomicUnit=on
  to rpy : MATLAB Function  TreatAsAtomicUnit=on
  roll : Outport
  pitch : Outport  Port=2
  yaw : Outport  Port=3
  WRB_matrix : Outport  Port=4
  wires:
  to rpy/2(pitch) -> pitch/1, to rotm/2(theta)
  to rotm/1(rotm) -> WRB_matrix/1  "WRB"
  to rpy/3(roll) -> roll/1, to rotm/3(phi)
  to rpy/1(yaw) -> to rotm/1(psi), yaw/1
  WRB/1 -> to rpy/1(rotation_matrix)

== system Quad_Tilt_Rotor_IdealModel/Subsystem21/Subsystem1 ==
  WRB : Inport
  to rotm : MATLAB Function  TreatAsAtomicUnit=on
  to rpy : MATLAB Function  TreatAsAtomicUnit=on
  roll : Outport
  pitch : Outport  Port=2
  yaw : Outport  Port=3
  WRB_matrix : Outport  Port=4
  wires:
  to rpy/2(pitch) -> pitch/1, to rotm/2(theta)
  to rotm/1(rotm) -> WRB_matrix/1  "WRB"
  to rpy/3(roll) -> roll/1, to rotm/3(phi)
  to rpy/1(yaw) -> to rotm/1(psi), yaw/1
  WRB/1 -> to rpy/1(rotation_matrix)

== system Quad_Tilt_Rotor_IdealModel/Subsystem9/Subsystem14 ==
  Angular_vel2 : Inport
  Abs : Abs
  Gain2 : Gain  Gain=[0;0;-Km]  Multiplication=Matrix(K*u) (u vector)
  Matrix Multiply : Product  Multiplication=Matrix(*)
  tauext2 : Outport
  wires:
  Angular_vel2/1 -> Abs/1, Matrix Multiply/1  "Angular_vel2"
  Abs/1 -> Matrix Multiply/2  "abs(Angular_vel2)"
  Gain2/1 -> tauext2/1
  Matrix Multiply/1 -> Gain2/1

== matlab function Quad_Tilt_Rotor_IdealModel/Subsystem4/MATLAB Function7 ==
  data: theta input; R output
function R = Rx(theta)

R = [1  0  0;
     0  cos(theta)  -sin(theta);
     0  sin(theta)   cos(theta)];

end

== matlab function Quad_Tilt_Rotor_IdealModel/Subsystem7/MATLAB Function10 ==
  data: theta input; R output
function R = Rz(theta)

R = [cos(theta)  -sin(theta)   0;
     sin(theta)   cos(theta)   0;
     0   0   1];

end

== matlab function Quad_Tilt_Rotor_IdealModel/Subsystem7/MATLAB Function11 ==
  data: theta input; R output
function R = Rx(theta)

R = [1  0  0;
     0  cos(theta)  -sin(theta);
     0  sin(theta)   cos(theta)];

end

== matlab function Quad_Tilt_Rotor_IdealModel/Subsystem8/MATLAB Function12 ==
  data: theta input; R output
function R = Rz(theta)

R = [cos(theta)  -sin(theta)   0;
     sin(theta)   cos(theta)   0;
     0   0   1];

end

== matlab function Quad_Tilt_Rotor_IdealModel/Subsystem8/MATLAB Function13 ==
  data: theta input; R output
function R = Rx(theta)

R = [1  0  0;
     0  cos(theta)  -sin(theta);
     0  sin(theta)   cos(theta)];

end

== matlab function Quad_Tilt_Rotor_IdealModel/Subsystem5/MATLAB Function14 ==
  data: theta input; R output
function R = Rz(theta)

R = [cos(theta)  -sin(theta)   0;
     sin(theta)   cos(theta)   0;
     0   0   1];

end

== matlab function Quad_Tilt_Rotor_IdealModel/Subsystem5/MATLAB Function15 ==
  data: theta input; R output
function R = Rx(theta)

R = [1  0  0;
     0  cos(theta)  -sin(theta);
     0  sin(theta)   cos(theta)];

end

== matlab function Quad_Tilt_Rotor_IdealModel/Subsystem6/MATLAB Function8 ==
  data: theta input; R output
function R = Rz(theta)

R = [cos(theta)  -sin(theta)   0;
     sin(theta)   cos(theta)   0;
     0   0   1];

end

== matlab function Quad_Tilt_Rotor_IdealModel/Subsystem6/MATLAB Function9 ==
  data: theta input; R output
function R = Rx(theta)

R = [1  0  0;
     0  cos(theta)  -sin(theta);
     0  sin(theta)   cos(theta)];

end

== matlab function Quad_Tilt_Rotor_IdealModel/Subsystem/MATLAB Function16 ==
  data: theta input; R output
function R = Rz(theta)

R = [cos(theta)  -sin(theta)   0;
     sin(theta)   cos(theta)   0;
     0   0   1];

end

== matlab function Quad_Tilt_Rotor_IdealModel/Subsystem/MATLAB Function17 ==
  data: theta input; R output
function R = Rx(theta)

R = [1  0  0;
     0  cos(theta)  -sin(theta);
     0  sin(theta)   cos(theta)];

end

== matlab function Quad_Tilt_Rotor_IdealModel/Subsystem/MATLAB Function18 ==
  data: theta input; R output
function R = Rz(theta)

R = [cos(theta)  -sin(theta)   0;
     sin(theta)   cos(theta)   0;
     0   0   1];

end

== matlab function Quad_Tilt_Rotor_IdealModel/Subsystem/MATLAB Function19 ==
  data: theta input; R output
function R = Rx(theta)

R = [1  0  0;
     0  cos(theta)  -sin(theta);
     0  sin(theta)   cos(theta)];

end

== matlab function Quad_Tilt_Rotor_IdealModel/Subsystem/MATLAB Function20 ==
  data: theta input; R output
function R = Rz(theta)

R = [cos(theta)  -sin(theta)   0;
     sin(theta)   cos(theta)   0;
     0   0   1];

end

== matlab function Quad_Tilt_Rotor_IdealModel/Subsystem/MATLAB Function21 ==
  data: theta input; R output
function R = Rx(theta)

R = [1  0  0;
     0  cos(theta)  -sin(theta);
     0  sin(theta)   cos(theta)];

end

== matlab function Quad_Tilt_Rotor_IdealModel/Subsystem/MATLAB Function22 ==
  data: theta input; R output
function R = Rz(theta)

R = [cos(theta)  -sin(theta)   0;
     sin(theta)   cos(theta)   0;
     0   0   1];

end

== matlab function Quad_Tilt_Rotor_IdealModel/Subsystem/MATLAB Function23 ==
  data: theta input; R output
function R = Rx(theta)

R = [1  0  0;
     0  cos(theta)  -sin(theta);
     0  sin(theta)   cos(theta)];

end

== matlab function Quad_Tilt_Rotor_IdealModel/MATLAB Function ==
  data: w input; hat output
function hat = skew(w)




hat = [ 0       -w(3)     w(2);
        w(3)     0       -w(1);
       -w(2)     w(1)     0];

== matlab function Quad_Tilt_Rotor_IdealModel/Subsystem15/MATLAB Function1 ==
  data: theta input; R output
function R = Rz(theta)

R = [cos(theta)  -sin(theta)   0;
     sin(theta)   cos(theta)   0;
     0   0   1];

end

== matlab function Quad_Tilt_Rotor_IdealModel/Subsystem15/MATLAB Function2 ==
  data: theta input; R output
function R = Rx(theta)

R = [1  0  0;
     0  cos(theta)  -sin(theta);
     0  sin(theta)   cos(theta)];

end

== matlab function Quad_Tilt_Rotor_IdealModel/Subsystem14/MATLAB Function3 ==
  data: theta input; R output
function R = Rz(theta)

R = [cos(theta)  -sin(theta)   0;
     sin(theta)   cos(theta)   0;
     0   0   1];

end

== matlab function Quad_Tilt_Rotor_IdealModel/Subsystem14/MATLAB Function4 ==
  data: theta input; R output
function R = Rx(theta)

R = [1  0  0;
     0  cos(theta)  -sin(theta);
     0  sin(theta)   cos(theta)];

end

== matlab function Quad_Tilt_Rotor_IdealModel/Subsystem13/MATLAB Function5 ==
  data: theta input; R output
function R = Rz(theta)

R = [cos(theta)  -sin(theta)   0;
     sin(theta)   cos(theta)   0;
     0   0   1];

end

== matlab function Quad_Tilt_Rotor_IdealModel/Subsystem13/MATLAB Function6 ==
  data: theta input; R output
function R = Rx(theta)

R = [1  0  0;
     0  cos(theta)  -sin(theta);
     0  sin(theta)   cos(theta)];

end

== matlab function Quad_Tilt_Rotor_IdealModel/Subsystem11/MATLAB Function7 ==
  data: theta input; R output
function R = Rz(theta)

R = [cos(theta)  -sin(theta)   0;
     sin(theta)   cos(theta)   0;
     0   0   1];

end

== matlab function Quad_Tilt_Rotor_IdealModel/Subsystem11/MATLAB Function8 ==
  data: theta input; R output
function R = Rx(theta)

R = [1  0  0;
     0  cos(theta)  -sin(theta);
     0  sin(theta)   cos(theta)];

end

== matlab function Quad_Tilt_Rotor_IdealModel/MATLAB Function1 ==
  data: omega1 input; angular_vel1 output; angular_vel2 output; angular_vel3 output; angular_vel4 output; omega2 input; omega3 input; omega4 input
function [angular_vel1,angular_vel2,angular_vel3,angular_vel4] = fcn(omega1,omega2,omega3,omega4)

angular_vel1 = sign(omega1) * sqrt(abs(omega1));
angular_vel2 = sign(omega2) * sqrt(abs(omega2));
angular_vel3 = sign(omega3) * sqrt(abs(omega3));
angular_vel4 = sign(omega4) * sqrt(abs(omega4));

== matlab function Quad_Tilt_Rotor_IdealModel/MATLAB Function2 ==
  data: WRB input; walpha1 output; walpha2 output; walpha3 output; walpha4 output; domega1 output; domega2 output; domega3 output; domega4 output; dWRB input; m input; IB input; L input; Kf input; Km input; alpha1 input; alpha2 input; alpha3 input; alpha4 input; omega1 input; omega2 input; omega3 input; omega4 input; dddpd input; ddpd input; dpd input; pd input; ddp input; dp input; p input; Rd input; ddwd input; dwd input; wd input; dwB input; wB input; inverse_result output; ToBeInversed output; RankBeforeInv output; eR output; eP output; RankJR output; RankRight output; attitude_phi input; attitude_theta input; attitude_psi input
function [walpha1,walpha2,walpha3,walpha4,domega1,domega2,domega3,domega4,inverse_result,ToBeInversed,RankBeforeInv,eR,eP,RankJR,RankRight] = fcn(WRB,dWRB,m,IB,L,Kf,Km,alpha1,alpha2,alpha3,alpha4,omega1,omega2,omega3,omega4,dddpd,ddpd,dpd,pd,ddp,dp,p,Rd,ddwd,dwd,wd,dwB,wB,attitude_phi,attitude_theta,attitude_psi)

omega= [omega1; omega2; omega3; omega4];

JR = [ 1/m * WRB                     [0  0  0; 0  0  0; 0  0  0];
       [0  0  0; 0  0  0; 0  0  0]   inv(IB)];
   
   
   
F = [       0             Kf*sin(alpha2)              0                -Kf*sin(alpha4);
       Kf*sin(alpha1)           0              -Kf*sin(alpha3)                 0;
      -Kf*cos(alpha1)     Kf*cos(alpha2)       -Kf*cos(alpha3)          Kf*cos(alpha4)]; 
   
tau = [        0        L*Kf*cos(alpha2)-Km*sin(alpha2)         0        -L*Kf*cos(alpha4)+Km*sin(alpha4);
        L*Kf*cos(alpha1)+Km*sin(alpha1)        0        -L*Kf*cos(alpha3)-Km*sin(alpha3)         0;
        L*Kf*sin(alpha1)-Km*cos(alpha1)   -L*Kf*sin(alpha2)-Km*cos(alpha2)   L*Kf*sin(alpha3)-Km*cos(alpha3)   -L*Kf*sin(alpha4)-Km*cos(alpha4)];
   
barJalpha = [F; tau];



sigmapart = [       0             Kf*cos(alpha2)              0                -Kf*cos(alpha4);
              Kf*cos(alpha1)           0              -Kf*cos(alpha3)                 0;
              Kf*sin(alpha1)     -Kf*sin(alpha2)       Kf*sin(alpha3)         -Kf*sin(alpha4)
                     0        -L*Kf*sin(alpha2)-Km*cos(alpha2)         0       L*Kf*sin(alpha4)+Km*cos(alpha4);
       -L*Kf*sin(alpha1)+Km*cos(alpha1)        0        L*Kf*sin(alpha3)-Km*cos(alpha3)         0;
        L*Kf*cos(alpha1)+Km*sin(alpha1)   -L*Kf*cos(alpha2)+Km*sin(alpha2)   L*Kf*cos(alpha3)+Km*sin(alpha3)   -L*Kf*cos(alpha4)+Km*sin(alpha4)] * diag([omega1,omega2,omega3,omega4]);

ToBeInversed = JR * [  barJalpha   sigmapart  ];

ToBeMinused = [ 1/m * dWRB * F * omega; [ 0; 0; 0]];




%% 


kp1 = 100 * diag([7.5,7.5,7.5]);        % 100 * diag([7.5,7.5,7.5])   (T = 0.0001); 100; 120

kp2 = 100 * diag([18.75,18.75,18.75]);   % 100 * diag([7.5,7.5,7.5])   (T = 0.0001); 100; 100

kp3 = 100 * diag([15.62,15.62,15.62]);  % 100 * diag([7.5,7.5,7.5])   (T = 0.0001); 100; 120



kw1 = 100 * diag([7.5,7.5,7.5]);          % 100 * diag([7.5,7.5,7.5])   (T = 0.0001);  100; 200

kw2 = 80 * diag([18.75,18.75,18.75]);     % 80 * diag([18.75,18.75,18.75]);  100; 160

kw3 = 165 * diag([15.62,15.62,15.62]);    % 165 * diag([15.62,15.62,15.62];  550; 165







dddpr = dddpd + kp1 * ( ddpd - ddp ) + kp2 * ( dpd - dp ) + kp3 * ( pd - p );




ToBeInvHat = WRB.' * Rd - Rd.' * WRB;

eR = 1/2 * [ ToBeInvHat(3,2) ; ToBeInvHat(1,3) ; ToBeInvHat(2,1) ];


ddwBr = ddwd + kw1 * ( dwd - dwB ) + kw2 * ( wd - wB ) + kw3 * eR;



eP = pd - p;


%%

result = pinv(ToBeInversed) * ( [dddpr ; ddwBr] - ToBeMinused );

walpha1 = result(5);
walpha2 = result(6);
walpha3 = result(7);
walpha4 = result(8);

domega1 = result(1);
domega2 = result(2);
domega3 = result(3);
domega4 = result(4);

inverse_result = pinv(ToBeInversed);

RankBeforeInv = rank(ToBeInversed);

RankJR = rank(JR);

RankRight = rank([  barJalpha   sigmapart  ]);

== matlab function Quad_Tilt_Rotor_IdealModel/Subsystem16/MATLAB Function3 ==
  data: w input; hat output
function hat = skew(w)




hat = [ 0       -w(3)     w(2);
        w(3)     0       -w(1);
       -w(2)     w(1)     0];

== matlab function Quad_Tilt_Rotor_IdealModel/Subsystem19/to rotm ==
  data: psi input; theta input; phi input; rotm output
function rotm = fcn(psi,theta,phi)

eul = [psi,theta,phi];


rotm = eul2rotm(eul);

== matlab function Quad_Tilt_Rotor_IdealModel/Subsystem19/to rpy ==
  data: yaw output; pitch output; rotation_matrix input; roll output
function [yaw,pitch,roll] = fcn(rotation_matrix)


eulZYX = rotm2eul(rotation_matrix);

yaw = eulZYX(1);

pitch = eulZYX(2);

roll = eulZYX(3);

== matlab function Quad_Tilt_Rotor_IdealModel/Subsystem20/MATLAB Function3 ==
  data: w input; hat output
function hat = skew(w)




hat = [ 0       -w(3)     w(2);
        w(3)     0       -w(1);
       -w(2)     w(1)     0];

== matlab function Quad_Tilt_Rotor_IdealModel/MATLAB Function4 ==
  data: vector input; skewed output
function skewed = skew(vector)


a = vector(1);
b = vector(2);
c = vector(3);

skewed = [ 0,  -c,  b;
           c,   0  -a;
          -b,  a,   0];

== matlab function Quad_Tilt_Rotor_IdealModel/Subsystem21/Subsystem1/to rotm ==
  data: psi input; theta input; phi input; rotm output
function rotm = fcn(psi,theta,phi)

eul = [psi,theta,phi];


rotm = eul2rotm(eul);

== matlab function Quad_Tilt_Rotor_IdealModel/Subsystem21/Subsystem1/to rpy ==
  data: yaw output; pitch output; rotation_matrix input; roll output
function [yaw,pitch,roll] = fcn(rotation_matrix)


eulZYX = rotm2eul(rotation_matrix);

yaw = eulZYX(1);

pitch = eulZYX(2);

roll = eulZYX(3);

== matlab function Quad_Tilt_Rotor_IdealModel/Subsystem21/MATLAB Function1 ==
  data: hat input; w output

function w = skew(hat)



w = [hat(3,2);hat(1,3);hat(2,1)];

== matlab function Quad_Tilt_Rotor_IdealModel/MATLAB Function3 ==
  data: theta input; R output
function R = Rx(theta)

R = [1  0  0;
     0  cos(theta)  -sin(theta);
     0  sin(theta)   cos(theta)];

end

== matlab function Quad_Tilt_Rotor_IdealModel/Subsystem20/Subsystem19/to rotm ==
  data: psi input; theta input; phi input; rotm output
function rotm = fcn(psi,theta,phi)

eul = [psi,theta,phi];


rotm = eul2rotm(eul);

== matlab function Quad_Tilt_Rotor_IdealModel/Subsystem20/Subsystem19/to rpy ==
  data: yaw output; pitch output; rotation_matrix input; roll output
function [yaw,pitch,roll] = fcn(rotation_matrix)


eulZYX = rotm2eul(rotation_matrix);

yaw = eulZYX(1);

pitch = eulZYX(2);

roll = eulZYX(3);

== matlab function Quad_Tilt_Rotor_IdealModel/Subsystem1/MATLAB Function1 ==
  data: theta input; R output
function R = Rx(theta)

R = [1  0  0;
     0  cos(theta)  -sin(theta);
     0  sin(theta)   cos(theta)];

end

== matlab function Quad_Tilt_Rotor_IdealModel/Subsystem1/MATLAB Function ==
  data: theta input; R output
function R = Rz(theta)

R = [cos(theta)  -sin(theta)   0;
     sin(theta)   cos(theta)   0;
     0   0   1];

end

== matlab function Quad_Tilt_Rotor_IdealModel/Subsystem2/MATLAB Function2 ==
  data: theta input; R output
function R = Rz(theta)

R = [cos(theta)  -sin(theta)   0;
     sin(theta)   cos(theta)   0;
     0   0   1];

end

== matlab function Quad_Tilt_Rotor_IdealModel/Subsystem2/MATLAB Function3 ==
  data: theta input; R output
function R = Rx(theta)

R = [1  0  0;
     0  cos(theta)  -sin(theta);
     0  sin(theta)   cos(theta)];

end

== matlab function Quad_Tilt_Rotor_IdealModel/Subsystem3/MATLAB Function4 ==
  data: theta input; R output
function R = Rz(theta)

R = [cos(theta)  -sin(theta)   0;
     sin(theta)   cos(theta)   0;
     0   0   1];

end

== matlab function Quad_Tilt_Rotor_IdealModel/Subsystem3/MATLAB Function5 ==
  data: theta input; R output
function R = Rx(theta)

R = [1  0  0;
     0  cos(theta)  -sin(theta);
     0  sin(theta)   cos(theta)];

end

== matlab function Quad_Tilt_Rotor_IdealModel/Subsystem4/MATLAB Function6 ==
  data: theta input; R output
function R = Rz(theta)

R = [cos(theta)  -sin(theta)   0;
     sin(theta)   cos(theta)   0;
     0   0   1];

end
